simulink model "distillation_demo"  (Simulink 6.0)
settings: Solver=ode45  StartTime=0.0  StopTime=100  RelTol=1e-3
PreLoadFcn:
  | load distillation_demo
undefined symbols (not defined in the file or in its folder): DiscIntNeverNeededParam, K1, K2, tau1, tau2
libraries: srolib x1, simulink x1
settings Model: Creator=pascal  LastModifiedBy=rlandy
settings DataIOCC: SignalLoggingName=DataLog
settings DebuggingCC: CheckExecutionContextPreStartOutputMsg=on  CheckExecutionContextRuntimeOutputMsg=on
settings ModelReferenceCC: UpdateModelReferenceTargets=IfOutOfDate
settings SFSimCC: SFSimApplyToAllLibs=on  SFSimBuildMode=Incremental

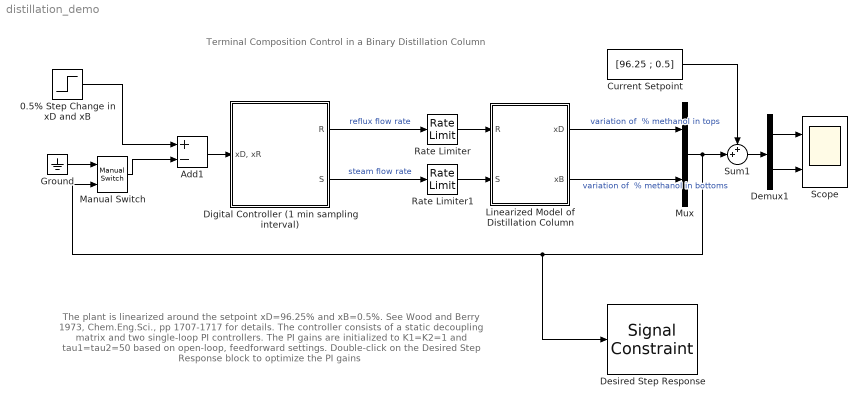
== system distillation_demo ==
  note: The plant is linearized around the setpoint xD=96.25% and xB=0.5%.
      | See Wood and Berry 1973, Chem.Eng.Sci., pp 1707-1717 for details.
      |
      | The controller consists of a static decoupling matrix and two
      | single-loop PI controllers. The PI gains are initialized to K1=K2=1
      | and tau1=tau2=50 based on open-loop, feedforward settings.
      |
      | Double-click on the Desired Step Response block
      | to optimize the PI gains
  note: Terminal Composition Control in a Binary Distillation Column
  0.5% Step Change in xD and xB : Step  Time=0  After=0.5  SampleTime=0
  Add1 : Sum  Inputs=+-  OutScaling=2^-10
  Current Setpoint : Constant  Value=[96.25 ; 0.5]  SampleTime=0
  Demux1 : Demux  Outputs=2
  Desired Step Response : srolib/Signal Constraint  DialogPosition=[0.040625 0.309166666666667 0.39 0.278333333333333]  SaveIn=workspace  SaveAs=distillation_optim  LogID=SRO_DataLog_1  Ylim=[-0.2 0.8]
  Digital Controller (1 min sampling interval) : Subsystem  PropExecContextAcrossSSBoundary=on
  Ground : Ground
  Linearized Model of Distillation Column : Subsystem  PropExecContextAcrossSSBoundary=on
  Manual Switch : simulink/Signal Routing/Manual Switch  sw=0  action=0
  Mux : Mux  Inputs=2
  Rate Limiter : RateLimiter  RisingSlewLimit=0.015  FallingSlewLimit=-0.015  SampleTimeMode=inherited
  Rate Limiter1 : RateLimiter  RisingSlewLimit=0.015  FallingSlewLimit=-0.015  SampleTimeMode=inherited
  Scope : Scope  NumInputPorts=2
      settings: YMin=-5~-5  YMax=5~5
  Sum1 : Sum  Inputs=++|
  wires:
  0.5% Step Change in xD and xB/1 -> Add1/1
  Digital Controller (1 min sampling interval)/1(R) -> Rate Limiter/1  "reflux flow rate"
  Digital Controller (1 min sampling interval)/2(S) -> Rate Limiter1/1  "steam flow rate"
  Linearized Model of Distillation Column/1(xD) -> Mux/1  "variation of  % methanol in tops"
  Linearized Model of Distillation Column/2(xB) -> Mux/2  "variation of  % methanol in bottoms"
  Mux/1 -> Manual Switch/2, Desired Step Response/1, Sum1/2
  Add1/1 -> Digital Controller (1 min sampling interval)/1("xD, xR  ")
  Demux1/1 -> Scope/1
  Demux1/2 -> Scope/2
  Manual Switch/1 -> Add1/2
  Ground/1 -> Manual Switch/1
  Rate Limiter/1 -> Linearized Model of Distillation Column/1("R  ")
  Rate Limiter1/1 -> Linearized Model of Distillation Column/2(S)
  Current Setpoint/1 -> Sum1/1
  Sum1/1 -> Demux1/1

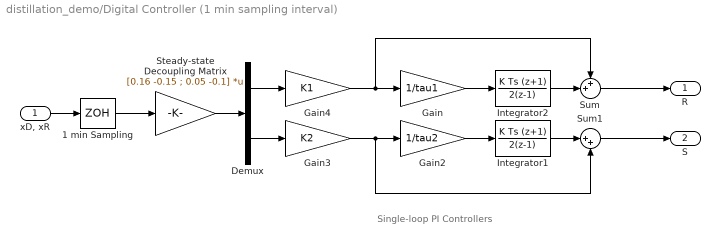
== system distillation_demo/Digital Controller (1 min sampling interval) ==
  note: Single-loop PI Controllers
  "xD, xR  " : Inport  LatchInput=off
  "1 min Sampling " : ZeroOrderHold
  Demux : Demux  Outputs=2
  Gain : Gain  Gain=1/tau1
  Gain2 : Gain  Gain=1/tau2
  Gain3 : Gain  Gain=K2
  Gain4 : Gain  Gain=K1
  Integrator1 : DiscreteIntegrator  IntegratorMethod=Integration: Trapezoidal  SaturateOnIntegerOverflow=on  ICPrevOutput=DiscIntNeverNeededParam  ICPrevScaledInput=DiscIntNeverNeededParam
  Integrator2 : DiscreteIntegrator  IntegratorMethod=Integration: Trapezoidal  SaturateOnIntegerOverflow=on  ICPrevOutput=DiscIntNeverNeededParam  ICPrevScaledInput=DiscIntNeverNeededParam
  Steady-state Decoupling Matrix : Gain  Gain=[0.16 -0.15 ; 0.05 -0.1]  Multiplication=Matrix(K*u)
  Sum : Sum  Inputs=++|
  Sum1 : Sum  Inputs=|++
  R : Outport
  S : Outport  Port=2
  wires:
  "xD, xR  "/1 -> "1 min Sampling "/1
  Steady-state Decoupling Matrix/1 -> Demux/1
  Demux/1 -> Gain4/1
  Gain/1 -> Integrator2/1
  Sum/1 -> R/1
  Demux/2 -> Gain3/1
  Integrator2/1 -> Sum/2
  Gain2/1 -> Integrator1/1
  Integrator1/1 -> Sum1/1
  Sum1/1 -> S/1
  "1 min Sampling "/1 -> Steady-state Decoupling Matrix/1
  Gain4/1 -> Gain/1, Sum/1
  Gain3/1 -> Gain2/1, Sum1/2

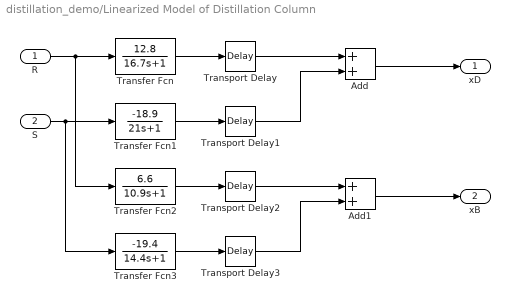
== system distillation_demo/Linearized Model of Distillation Column ==
  "R  " : Inport  LatchInput=off
  S : Inport  Port=2  LatchInput=off
  Add : Sum  OutScaling=2^-10
  Add1 : Sum  OutScaling=2^-10
  Transfer Fcn : TransferFcn  Numerator=12.8  Denominator=[16.7 1]
  Transfer Fcn1 : TransferFcn  Numerator=-18.9  Denominator=[21 1]
  Transfer Fcn2 : TransferFcn  Numerator=6.6  Denominator=[10.9 1]
  Transfer Fcn3 : TransferFcn  Numerator=-19.4  Denominator=[14.4 1]
  Transport Delay : TransportDelay
  Transport Delay1 : TransportDelay  DelayTime=3
  Transport Delay2 : TransportDelay  DelayTime=7
  Transport Delay3 : TransportDelay  DelayTime=3
  xD : Outport
  xB : Outport  Port=2
  wires:
  "R  "/1 -> Transfer Fcn/1, Transfer Fcn2/1
  Transfer Fcn/1 -> Transport Delay/1
  Transport Delay/1 -> Add/1
  Add/1 -> xD/1
  S/1 -> Transfer Fcn1/1, Transfer Fcn3/1
  Transfer Fcn1/1 -> Transport Delay1/1
  Transport Delay1/1 -> Add/2
  Transfer Fcn2/1 -> Transport Delay2/1
  Transport Delay2/1 -> Add1/1
  Add1/1 -> xB/1
  Transfer Fcn3/1 -> Transport Delay3/1
  Transport Delay3/1 -> Add1/2
